simulink model "coaxialQuad_model"  (R2022a)
settings: Solver=VariableStepAuto  StartTime=0.0  StopTime=40  RelTol=1e-3
values from neighbouring files (symbols this model uses):
  Ah = 5,8    [coaxialQuad_init.m]
  Ax = 0    [coaxialQuad_init.m]
  Ay = 0    [coaxialQuad_init.m]
  b = 1.869E-7    (= 1.869e-07)    [coaxialQuad_init.m]
  b_m = 2.415e-6    (= 2.415e-06)    [coaxialQuad_init.m]
  C = 45    [coaxialQuad_init.m]
  d = 1.706E-8    (= 1.706e-08)    [coaxialQuad_init.m]
  Ixx = 0.182    [coaxialQuad_init.m]
  Iyy = 0.188    [coaxialQuad_init.m]
  Izz = 0.335    [coaxialQuad_init.m]
  J = 6.5e-7    (= 6.5e-07)    [coaxialQuad_init.m]
  K_emf = 0.00255    [coaxialQuad_init.m]
  Kt = 0.00255    [coaxialQuad_init.m]
  l = 0.1    [coaxialQuad_init.m]
  L = 1.17e-4    (= 0.000117)    [coaxialQuad_init.m]
  m = 3.1    [coaxialQuad_init.m]
  omega_max = inf    [coaxialQuad_init.m]
  omega_min = 0    [coaxialQuad_init.m]
  phi_D = 0.1    [coaxialQuad_init.m]
  phi_I = 2    [coaxialQuad_init.m]
  phi_P = 2    [coaxialQuad_init.m]
  psi_D = 0    [coaxialQuad_init.m]
  psi_I = 0.1    [coaxialQuad_init.m]
  psi_P = 0.1    [coaxialQuad_init.m]
  R = 0.117    [coaxialQuad_init.m]
  theta_D = 0.1    [coaxialQuad_init.m]
  theta_I = 2    [coaxialQuad_init.m]
  theta_P = 2    [coaxialQuad_init.m]
  V = 16.8    [coaxialQuad_init.m]
  Z_D = 10    [coaxialQuad_init.m]
  Z_I = 5    [coaxialQuad_init.m]
  Z_P = 10    [coaxialQuad_init.m]
undefined symbols (not defined in the file or in its folder): Ion, Lithium
libraries: simulink x17, spsBatteryLib x1, spsControlledCurrentSourceLib x1, spspowerguiLib x1
settings Model: Creator=furkan  LastModifiedBy=Neo
settings DebuggingCC: AlgebraicLoopMsg=none  UnconnectedInputMsg=warning  UnconnectedOutputMsg=warning  UnconnectedLineMsg=warning
settings RTWCC: DLArmComputeVersion=19.05

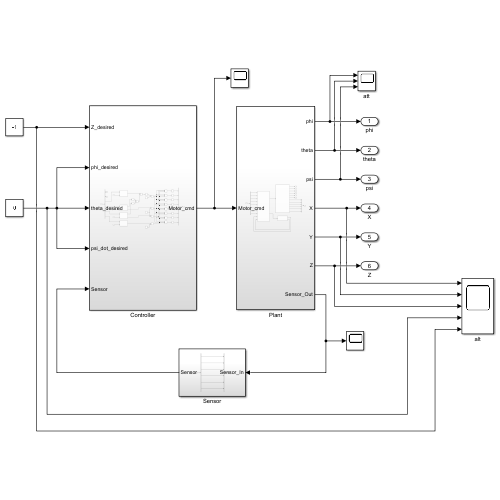
[thumbnail: Simulink's stored preview of the top-level diagram]
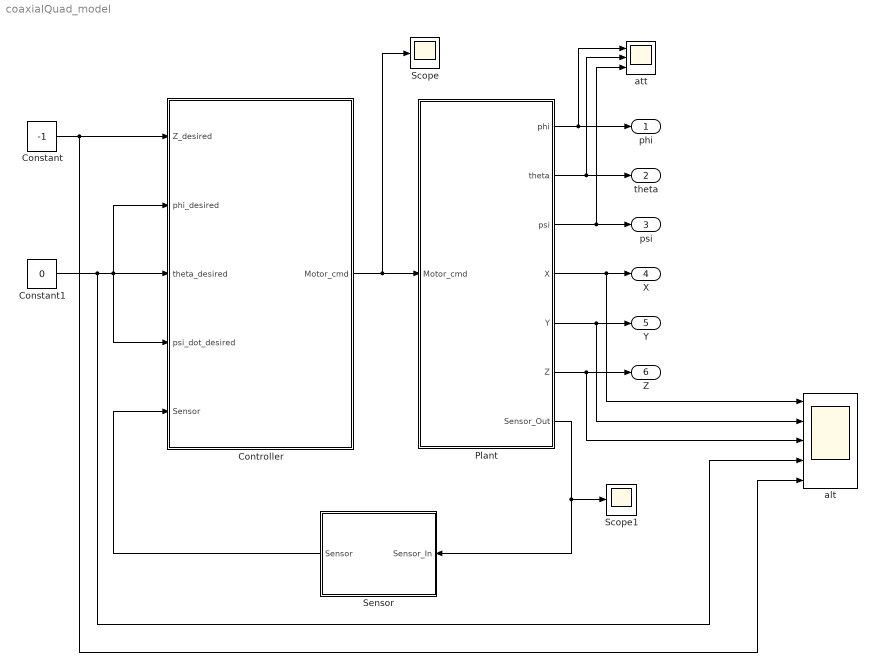
== system coaxialQuad_model ==
  Constant : Constant  Value=-1
  Constant1 : Constant  Value=0
  Controller : Subsystem
  Plant : Subsystem
  Scope : Scope
  Scope1 : Scope
  Sensor : Subsystem
  alt : Scope  NumInputPorts=5
  att : Scope  NumInputPorts=3
  phi : Outport
  theta : Outport  Port=2
  psi : Outport  Port=3
  X : Outport  Port=4
  Y : Outport  Port=5
  Z : Outport  Port=6
  wires:
  Plant/1(phi) -> phi/1, att/1
  Plant/2(theta) -> theta/1, att/2
  Plant/3(psi) -> att/3, psi/1
  Plant/4(X) -> X/1, alt/1
  Plant/5(Y) -> Y/1, alt/2
  Plant/6(Z) -> Z/1, alt/3
  Constant/1 -> Controller/1(Z_desired), alt/5
  Constant1/1 -> Controller/3(theta_desired), Controller/2(phi_desired), Controller/4(psi_dot_desired), alt/4
  Plant/7(Sensor_Out) -> Scope1/1, Sensor/1(Sensor_In)
  Sensor/1(Sensor) -> Controller/5(Sensor)
  Controller/1(Motor_cmd) -> Scope/1, Plant/1(Motor_cmd)

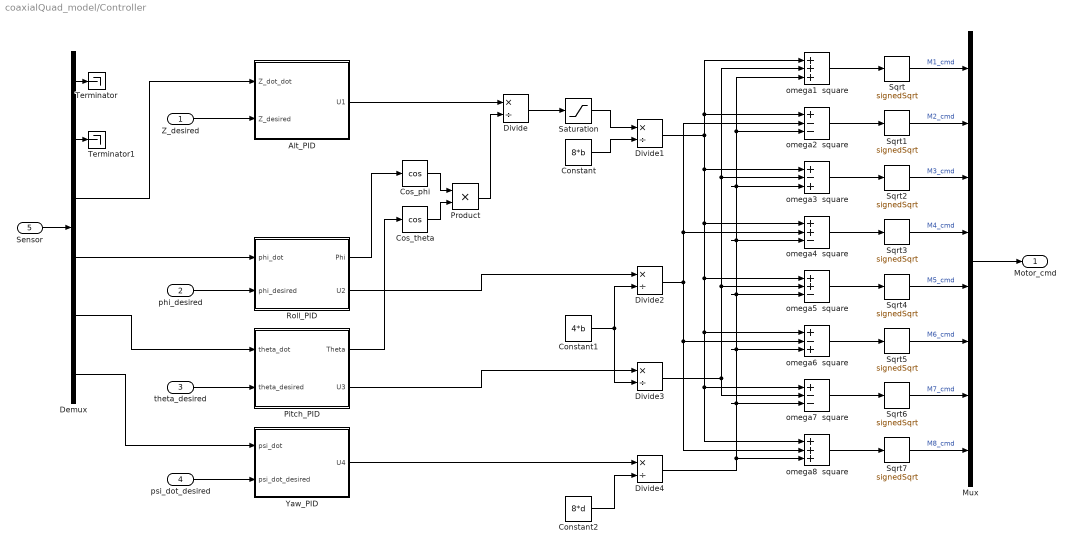
== system coaxialQuad_model/Controller ==
  Z_desired : Inport
  phi_desired : Inport  Port=2
  theta_desired : Inport  Port=3
  psi_dot_desired : Inport  Port=4
  Sensor : Inport  Port=5
  Alt_PID : Subsystem
  Constant : Constant  Value=8*b
  Constant1 : Constant  Value=4*b
  Constant2 : Constant  Value=8*d
  Cos_phi : Trigonometry  Operator=cos
  Cos_theta : Trigonometry  Operator=cos
  Demux : Demux  Outputs=6
  Divide{,1..4} (5 alike) : Product  Inputs=*/  RndMeth=Zero  SaturateOnIntegerOverflow=on
  Mux : Mux  Inputs=8
  Pitch_PID : Subsystem
  Product : Product
  Roll_PID : Subsystem
  Saturation : Saturate  UpperLimit=inf  LowerLimit=0
  Sqrt{,1..7} (8 alike) : Sqrt  Operator=signedSqrt
  Terminator : Terminator
  Terminator1 : Terminator
  Yaw_PID : Subsystem
  omega1  square : Sum  Inputs=+++
  omega2  square : Sum  Inputs=+--
  omega3  square : Sum  Inputs=+-+
  omega4  square : Sum  Inputs=++-
  omega5  square : Sum  Inputs=++-
  omega6  square : Sum  Inputs=+-+
  omega7  square : Sum  Inputs=+--
  omega8  square : Sum  Inputs=+++
  Motor_cmd : Outport
  wires:
  Cos_phi/1 -> Product/1
  Cos_theta/1 -> Product/2
  Product/1 -> Divide/2
  Demux/3 -> Alt_PID/1(Z_dot_dot)
  Z_desired/1 -> Alt_PID/2(Z_desired)
  Alt_PID/1(U1) -> Divide/1
  Divide/1 -> Saturation/1
  Constant/1 -> Divide1/2
  Saturation/1 -> Divide1/1
  Constant1/1 -> Divide3/2, Divide2/2
  Constant2/1 -> Divide4/2
  Demux/4 -> Roll_PID/1(phi_dot)
  phi_desired/1 -> Roll_PID/2(phi_desired)
  Roll_PID/2(U2) -> Divide2/1
  Demux/5 -> Pitch_PID/1(theta_dot)
  theta_desired/1 -> Pitch_PID/2(theta_desired)
  Pitch_PID/2(U3) -> Divide3/1
  Demux/6 -> Yaw_PID/1(psi_dot)
  psi_dot_desired/1 -> Yaw_PID/2(psi_dot_desired)
  Yaw_PID/1(U4) -> Divide4/1
  Divide1/1 -> omega2  square/1, omega1  square/1, omega3  square/1, omega4  square/1, omega5  square/1, omega6  square/1, omega7  square/1, omega8  square/1
  Divide3/1 -> omega7  square/2, omega5  square/2, omega3  square/2, omega1  square/2
  Divide4/1 -> omega8  square/3, omega7  square/3, omega6  square/3, omega5  square/3, omega4  square/3, omega3  square/3, omega1  square/3, omega2  square/3
  omega1  square/1 -> Sqrt/1
  Sqrt/1 -> Mux/1  "M1_cmd"
  Sqrt1/1 -> Mux/2  "M2_cmd"
  omega2  square/1 -> Sqrt1/1
  omega4  square/1 -> Sqrt3/1
  Sqrt3/1 -> Mux/4  "M4_cmd"
  Sqrt2/1 -> Mux/3  "M3_cmd"
  omega3  square/1 -> Sqrt2/1
  omega7  square/1 -> Sqrt6/1
  Sqrt6/1 -> Mux/7  "M7_cmd"
  Sqrt7/1 -> Mux/8  "M8_cmd"
  omega8  square/1 -> Sqrt7/1
  omega6  square/1 -> Sqrt5/1
  Sqrt5/1 -> Mux/6  "M6_cmd"
  Sqrt4/1 -> Mux/5  "M5_cmd"
  omega5  square/1 -> Sqrt4/1
  Divide2/1 -> omega8  square/2, omega6  square/2, omega2  square/2, omega4  square/2
  Demux/1 -> Terminator/1
  Demux/2 -> Terminator1/1
  Sensor/1 -> Demux/1
  Roll_PID/1(Phi) -> Cos_phi/1
  Pitch_PID/1(Theta) -> Cos_theta/1
  Mux/1 -> Motor_cmd/1

== system coaxialQuad_model/Plant ==
  Motor_cmd : Inport
  Battery Plant : Subsystem
  Body Plant : Subsystem
  Demux : Demux  Outputs=8
  Motor Plant : Subsystem
  Mux : Mux  Inputs=6
  phi : Outport
  theta : Outport  Port=2
  psi : Outport  Port=3
  X : Outport  Port=4
  Y : Outport  Port=5
  Z : Outport  Port=6
  Sensor_Out : Outport  Port=7
  wires:
  Body Plant/2(theta) -> theta/1
  Demux/7 -> Motor Plant/7(M7_cmd)  "M7_cmd"
  Demux/1 -> Motor Plant/1(M1_cmd)  "M1_cmd"
  Body Plant/3(psi) -> psi/1
  Body Plant/1(phi) -> phi/1
  Demux/5 -> Motor Plant/5(M5_cmd)  "M5_cmd"
  Demux/2 -> Motor Plant/2(M2_cmd)  "M2_cmd"
  Body Plant/4(X) -> X/1
  Demux/8 -> Motor Plant/8(M8_cmd)  "M8_cmd"
  Body Plant/5(Y) -> Y/1
  Demux/4 -> Motor Plant/4(M4_cmd)  "M4_cmd"
  Body Plant/6(Z) -> Z/1
  Battery Plant/1(Aval_Current) -> Motor Plant/9(Aval_Current)
  Battery Plant/2(Voltage) -> Motor Plant/10(Voltage)
  Demux/6 -> Motor Plant/6(M6_cmd)  "M6_cmd"
  Motor Plant/2(Current) -> Battery Plant/1(Current_draw)
  Demux/3 -> Motor Plant/3(M3_cmd)  "M3_cmd"
  Body Plant/7(X_dot_dot) -> Mux/1  "X_dot_dot"
  Body Plant/8(Y_dot_dot) -> Mux/2  "Y_dot_dot"
  Body Plant/9(Z_dot_dot) -> Mux/3  "Z_dot_dot"
  Body Plant/11(theta_dot) -> Mux/5  "theta_dot"
  Body Plant/12(psi_dot) -> Mux/6  "psi_dot"
  Body Plant/10(phi_dot) -> Mux/4  "phi_dot"
  Mux/1 -> Sensor_Out/1
  Motor_cmd/1 -> Demux/1
  Motor Plant/1(Omegas) -> Body Plant/1(omegas)

== system coaxialQuad_model/Sensor ==
  Sensor_In : Inport
  Demux : Demux  Outputs=6
  Mux : Mux  Inputs=6
  Sensor : Outport
  wires:
  Demux/2 -> Mux/2  "Y_dot_dot"
  Demux/3 -> Mux/3  "Z_dot_dot"
  Demux/6 -> Mux/6  "psi_dot"
  Demux/5 -> Mux/5  "theta_dot"
  Demux/4 -> Mux/4  "phi_dot"
  Demux/1 -> Mux/1  "X_dot_dot"
  Sensor_In/1 -> Demux/1
  Mux/1 -> Sensor/1

== system coaxialQuad_model/Controller/Alt_PID ==
  Z_dot_dot : Inport
  Z_desired : Inport  Port=2
  Add : Sum  Inputs=+-
  Add1 : Sum  Inputs=++-
  Integrator : Integrator
  Integrator1 : Integrator  LimitOutput=on  UpperSaturationLimit=0
  Integrator2 : Integrator
  Z_D : Gain  Gain=Z_D
  Z_I : Gain  Gain=Z_I
  Z_P : Gain  Gain=Z_P
  U1 : Outport
  wires:
  Integrator1/1 -> Add/2
  Z_dot_dot/1 -> Integrator/1
  Z_desired/1 -> Add/1
  Integrator/1 -> Z_D/1, Integrator1/1
  Add/1 -> Z_P/1, Integrator2/1
  Z_I/1 -> Add1/2
  Integrator2/1 -> Z_I/1
  Z_D/1 -> Add1/3
  Z_P/1 -> Add1/1
  Add1/1 -> U1/1

== system coaxialQuad_model/Controller/Pitch_PID ==
  theta_dot : Inport
  theta_desired : Inport  Port=2
  Add4 : Sum  Inputs=+-
  Add5 : Sum  Inputs=++-
  Integrator5 : Integrator  WrapState=on
  Integrator6 : Integrator
  Theta_D : Gain  Gain=theta_D
  Theta_I : Gain  Gain=theta_I
  Theta_P : Gain  Gain=theta_P
  Theta : Outport
  U3 : Outport  Port=2
  wires:
  Theta_D/1 -> Add5/3
  Theta_I/1 -> Add5/2
  theta_dot/1 -> Theta_D/1, Integrator5/1
  Integrator5/1 -> Theta/1, Add4/2
  Add4/1 -> Integrator6/1, Theta_P/1
  Theta_P/1 -> Add5/1
  theta_desired/1 -> Add4/1
  Integrator6/1 -> Theta_I/1
  Add5/1 -> U3/1

== system coaxialQuad_model/Controller/Roll_PID ==
  phi_dot : Inport
  phi_desired : Inport  Port=2
  Add2 : Sum  Inputs=+-
  Add3 : Sum  Inputs=++-
  Integrator3 : Integrator  WrapState=on
  Integrator4 : Integrator
  Phi_D : Gain  Gain=phi_D
  Phi_I : Gain  Gain=phi_I
  Phi_P : Gain  Gain=phi_P
  Phi : Outport
  U2 : Outport  Port=2
  wires:
  phi_desired/1 -> Add2/1
  Integrator3/1 -> Phi/1, Add2/2
  phi_dot/1 -> Phi_D/1, Integrator3/1
  Integrator4/1 -> Phi_I/1
  Add2/1 -> Phi_P/1, Integrator4/1
  Phi_P/1 -> Add3/1
  Phi_I/1 -> Add3/2
  Add3/1 -> U2/1
  Phi_D/1 -> Add3/3

== system coaxialQuad_model/Controller/Yaw_PID ==
  psi_dot : Inport
  psi_dot_desired : Inport  Port=2
  Add6 : Sum  Inputs=-+
  Add7 : Sum  Inputs=+++
  Derivative : Derivative
  Integrator7 : Integrator
  Psi_D : Gain  Gain=psi_D
  Psi_I : Gain  Gain=psi_I
  Psi_P : Gain  Gain=psi_P
  U4 : Outport
  wires:
  Psi_D/1 -> Add7/3
  Psi_I/1 -> Add7/2
  Integrator7/1 -> Psi_I/1
  psi_dot_desired/1 -> Add6/2
  Psi_P/1 -> Add7/1
  Add6/1 -> Derivative/1, Psi_P/1, Integrator7/1
  Derivative/1 -> Psi_D/1
  psi_dot/1 -> Add6/1
  Add7/1 -> U4/1

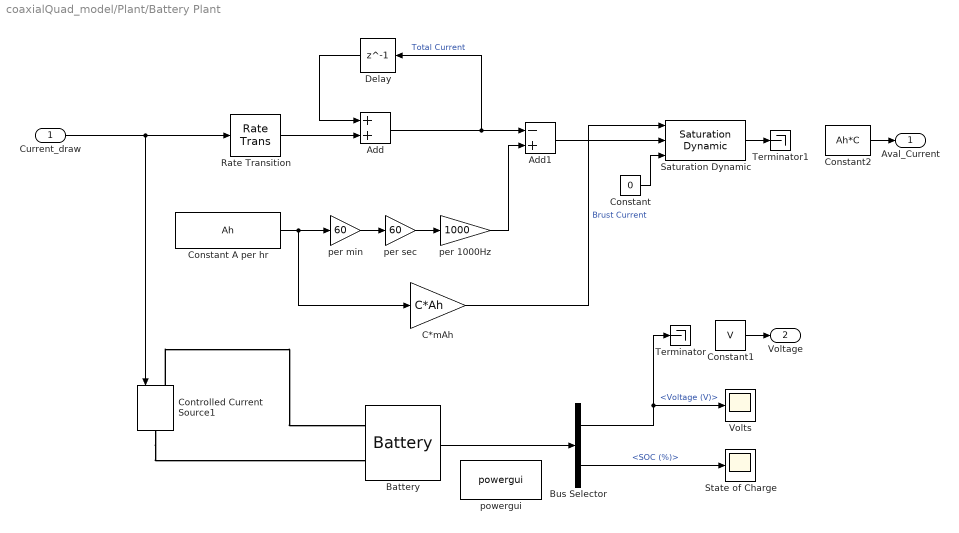
== system coaxialQuad_model/Plant/Battery Plant ==
  Current_draw : Inport
  Add : Sum
  Add1 : Sum  Inputs=-+
  Battery : spsBatteryLib/Battery  BatType=Lithium-Ion  ShowTempParam=off  ThermalPreset=no  ShowAgeParam=off  NomV=V  NomQ=Ah  SOC=100  Batt_Tr=1  PresetModel=on  MaxQ=5  MinV=12.6  FullV=19.555  Dis_rate=2.1739  R=0.0336  Normal_OP=4.5217  expZone="[18.1505     0.245652]"  current=[6.5 13 32.5]  Units=Time  Tci=20  NomT=20  T2=-30  MaxQ2=4.8  FullV2=7.1  Normal_OP2=5.655  expZone2="[6.58           1]"  Rca=0.6  ti=2000  Dp=0  Neq0=0  Tsim=1e6  Ta1=25  Qeol=5.4*0.9  Reol=0.013333*1.2  Char_age=[2.3478, 3]  Dis_age=[2.3478, 10]  N1=1500  N2=10500  N3=1000  N4=1400  Ta2=45  N5=950
  Bus Selector : BusSelector  OutputSignals=Voltage (V),SOC (%)
  C*mAh : Gain  Gain=C*Ah
  Constant : Constant  Value=0
  Constant A per hr : Constant  Value=Ah
  Constant1 : Constant  Value=V
  Constant2 : Constant  Value=Ah*C
  Controlled Current Source1 : spsControlledCurrentSourceLib/Controlled Current Source  Initialize=on  Source_Type=DC  Amplitude=0  Phase=0  Frequency=0  Measurements=None
  Delay : Delay  DelayLength=1
  Rate Transition : RateTransition
  Saturation Dynamic : simulink/Discontinuities/Saturation Dynamic  OutMin=[]  OutMax=[]  OutDataTypeStr=Inherit: Same as second input  OutDataType=fixdt(1, 16)  OutScaling=2^-10  DoSatur=off
  State of Charge : Scope
  Terminator : Terminator
  Terminator1 : Terminator
  Volts : Scope
  per 1000Hz : Gain  Gain=1000
  per min : Gain  Gain=60
  per sec : Gain  Gain=60
  powergui : spspowerguiLib/powergui  Priority=1  SimulationMode=Discrete  SampleTime=0.001  frequency=60  Iterations=50  frequencyindice=0  Pbase=100e6  ErrMax=1e-4  UnitsV=kV  UnitsW=MW  buscounter=0  FunctionMessages=off  echomessages=off  EnableUseOfTLC=off  CurrentSourceSwitches=off  DisableSnubberDevices=off  DisableRonSwitches=off  DisableVfSwitches=off  DisplayEquations=off  AutomaticDiscreteSolvers=off  SolverType=Tustin/Backward Euler (TBE)  Interpol=off  ExternalGateDelay=off  methode=off  Ts=100  x0status=blocks  SPID=on  SwTol=0  HookPort=off  NonlinearTolerance=1e-4  nMaxIteration=100  ContinueOnMaxIteration=off  RestoreLinks=warning  ResistiveCurrentMeasurement=off  Frange=[0:2:500]  Ylog=off  Xlog=on  ShowGrid=off  save=off  variable=ZData  structure=0  ZoomFFT=off  StartTime=0.0  cycles=1  DisplayStyle=1  fundamental=60  FreqAxis=off  MaxFrequency=1000  frequencyindicesteady=1  RmsSteady=1  display=off
  Aval_Current : Outport
  Voltage : Outport  Port=2
  wires:
  Current_draw/1 -> Controlled Current Source1/1, Rate Transition/1
  Rate Transition/1 -> Add/2
  Delay/1 -> Add/1
  Add/1 -> Add1/1, Delay/1  "Total Current"
  Constant A per hr/1 -> C*mAh/1, per min/1
  per min/1 -> per sec/1
  per sec/1 -> per 1000Hz/1
  per 1000Hz/1 -> Add1/2
  Add1/1 -> Saturation Dynamic/2
  C*mAh/1 -> Saturation Dynamic/1  "Brust Current"
  Constant/1 -> Saturation Dynamic/3
  Bus Selector/1 -> Terminator/1, Volts/1  "<Voltage (V)>"
  Bus Selector/2 -> State of Charge/1  "<SOC (%)>"
  Battery/1 -> Bus Selector/1
  Constant2/1 -> Aval_Current/1
  Saturation Dynamic/1 -> Terminator1/1
  Constant1/1 -> Voltage/1
  connections:
  Controlled Current Source1/RConn1 -- Battery/LConn2
  Controlled Current Source1/LConn1 -- Battery/LConn1

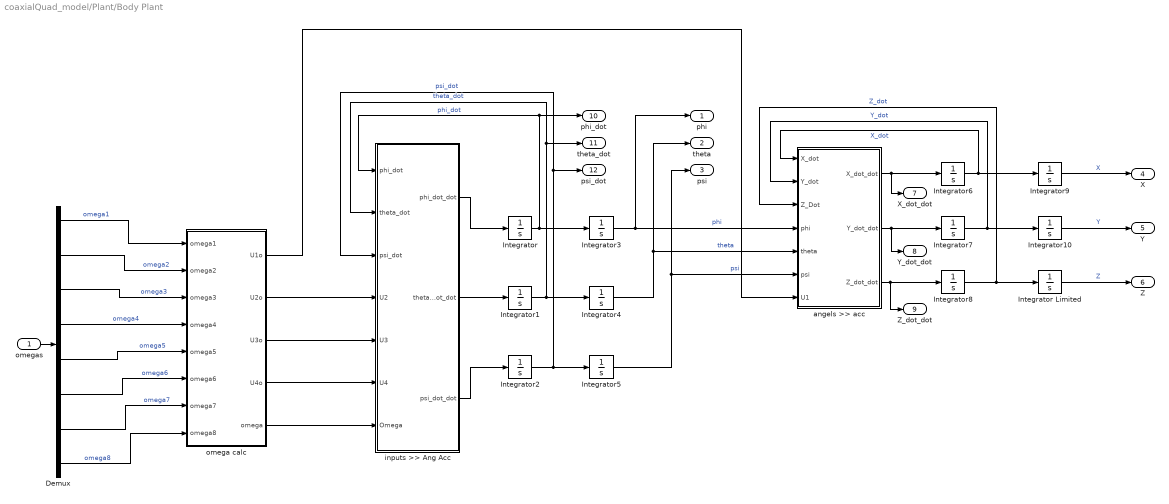
== system coaxialQuad_model/Plant/Body Plant ==
  omegas : Inport
  Demux : Demux  Outputs=8
  Integrator{,1..2,6..10} (8 alike) : Integrator
  Integrator Limited : Integrator  LimitOutput=on  UpperSaturationLimit=0
  Integrator3 : Integrator  WrapState=on
  Integrator4 : Integrator  WrapState=on
  Integrator5 : Integrator  WrapState=on
  angels >> acc : Subsystem
  inputs >> Ang Acc : Subsystem
  omega calc : Subsystem
  phi : Outport
  theta : Outport  Port=2
  psi : Outport  Port=3
  X : Outport  Port=4
  Y : Outport  Port=5
  Z : Outport  Port=6
  X_dot_dot : Outport  Port=7
  Y_dot_dot : Outport  Port=8
  Z_dot_dot : Outport  Port=9
  phi_dot : Outport  Port=10
  theta_dot : Outport  Port=11
  psi_dot : Outport  Port=12
  wires:
  Integrator5/1 -> psi/1, angels >> acc/6(psi)  "psi"
  omega calc/1(U1o) -> angels >> acc/7(U1)
  angels >> acc/1(X_dot_dot) -> X_dot_dot/1, Integrator6/1
  Integrator1/1 -> Integrator4/1, inputs >> Ang Acc/2(theta_dot), theta_dot/1  "theta_dot"
  Integrator2/1 -> Integrator5/1, inputs >> Ang Acc/3(psi_dot), psi_dot/1  "psi_dot"
  Demux/4 -> omega calc/4(omega4)  "omega4"
  Integrator4/1 -> theta/1, angels >> acc/5(theta)  "theta"
  angels >> acc/2(Y_dot_dot) -> Y_dot_dot/1, Integrator7/1
  Demux/6 -> omega calc/6(omega6)  "omega6"
  Integrator10/1 -> Y/1  "Y"
  angels >> acc/3(Z_dot_dot) -> Z_dot_dot/1, Integrator8/1
  Integrator3/1 -> phi/1, angels >> acc/4(phi)  "phi"
  Integrator/1 -> Integrator3/1, inputs >> Ang Acc/1(phi_dot), phi_dot/1  "phi_dot"
  Integrator6/1 -> angels >> acc/1(X_dot), Integrator9/1  "X_dot"
  Demux/2 -> omega calc/2(omega2)  "omega2"
  Integrator Limited/1 -> Z/1  "Z"
  inputs >> Ang Acc/3(psi_dot_dot) -> Integrator2/1
  omega calc/5(omega) -> inputs >> Ang Acc/7(Omega)
  Integrator9/1 -> X/1  "X"
  Integrator8/1 -> Integrator Limited/1, angels >> acc/3(Z_Dot)  "Z_dot"
  Integrator7/1 -> Integrator10/1, angels >> acc/2(Y_dot)  "Y_dot"
  inputs >> Ang Acc/1(phi_dot_dot) -> Integrator/1
  Demux/7 -> omega calc/7(omega7)  "omega7"
  omega calc/4(U4o) -> inputs >> Ang Acc/6(U4)
  omega calc/2(U2o) -> inputs >> Ang Acc/4(U2)
  Demux/8 -> omega calc/8(omega8)  "omega8"
  omega calc/3(U3o) -> inputs >> Ang Acc/5(U3)
  Demux/5 -> omega calc/5(omega5)  "omega5"
  Demux/3 -> omega calc/3(omega3)  "omega3"
  Demux/1 -> omega calc/1(omega1)  "omega1"
  inputs >> Ang Acc/2(theta_dot_dot) -> Integrator1/1
  omegas/1 -> Demux/1

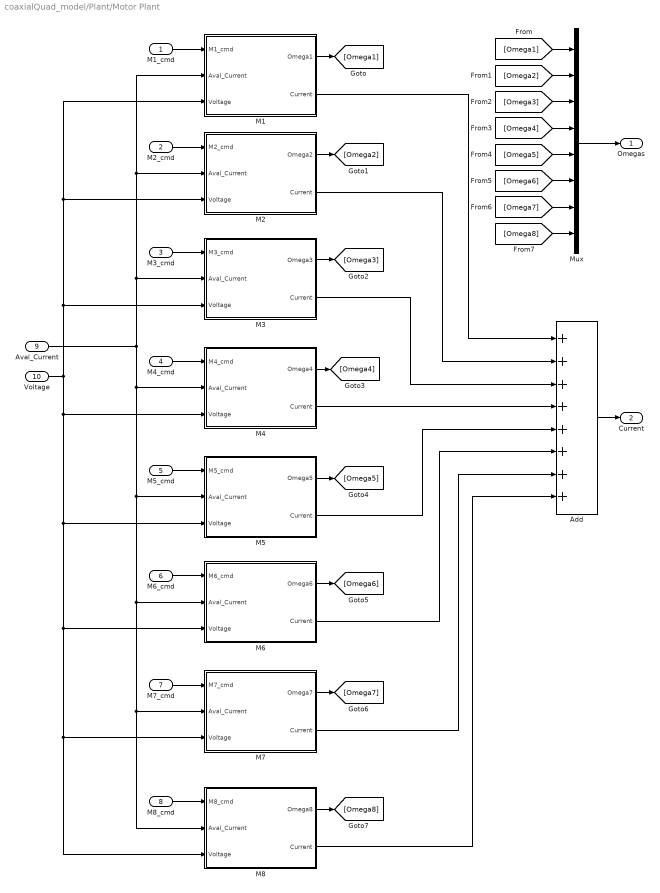
== system coaxialQuad_model/Plant/Motor Plant ==
  M1_cmd : Inport
  M2_cmd : Inport  Port=2
  M3_cmd : Inport  Port=3
  M4_cmd : Inport  Port=4
  M5_cmd : Inport  Port=5
  M6_cmd : Inport  Port=6
  M7_cmd : Inport  Port=7
  M8_cmd : Inport  Port=8
  Aval_Current : Inport  Port=9
  Voltage : Inport  Port=10
  Add : Sum  Inputs=++++++++
  M1 : Subsystem
  M2 : Subsystem
  M3 : Subsystem
  M4 : Subsystem
  M5 : Subsystem
  M6 : Subsystem
  M7 : Subsystem
  M8 : Subsystem
  Mux : Mux  Inputs=8
  Omegas : Outport
  Current : Outport  Port=2
  wires:
  M1_cmd/1 -> M1/1(M1_cmd)
  M2_cmd/1 -> M2/1(M2_cmd)
  M3_cmd/1 -> M3/1(M3_cmd)
  M4_cmd/1 -> M4/1(M4_cmd)
  M6_cmd/1 -> M6/1(M6_cmd)
  Voltage/1 -> M4/3(Voltage), M6/3(Voltage), M7/3(Voltage), M8/3(Voltage), M5/3(Voltage), M1/3(Voltage), M2/3(Voltage), M3/3(Voltage)
  Aval_Current/1 -> M2/2(Aval_Current), M1/2(Aval_Current), M3/2(Aval_Current), M7/2(Aval_Current), M8/2(Aval_Current), M6/2(Aval_Current), M5/2(Aval_Current), M4/2(Aval_Current)
  M8_cmd/1 -> M8/1(M8_cmd)
  M5_cmd/1 -> M5/1(M5_cmd)
  M7_cmd/1 -> M7/1(M7_cmd)
  M1/2(Current) -> Add/1
  M2/2(Current) -> Add/2
  M3/2(Current) -> Add/3
  M4/2(Current) -> Add/4
  M5/2(Current) -> Add/5
  M6/2(Current) -> Add/6
  M7/2(Current) -> Add/7
  M8/2(Current) -> Add/8
  Add/1 -> Current/1
  Mux/1 -> Omegas/1
  M1/1(Omega1) -> [Omega1]
  M2/1(Omega2) -> [Omega2]
  M3/1(Omega3) -> [Omega3]
  M8/1(Omega8) -> [Omega8]
  M7/1(Omega7) -> [Omega7]
  M5/1(Omega5) -> [Omega5]
  M6/1(Omega6) -> [Omega6]
  M4/1(Omega4) -> [Omega4]
  [Omega1] -> Mux/1
  [Omega2] -> Mux/2
  [Omega3] -> Mux/3
  [Omega4] -> Mux/4
  [Omega5] -> Mux/5
  [Omega6] -> Mux/6
  [Omega7] -> Mux/7
  [Omega8] -> Mux/8

== system coaxialQuad_model/Plant/Body Plant/angels >> acc ==
  X_dot : Inport
  Y_dot : Inport  Port=2
  Z_Dot : Inport  Port=3
  phi : Inport  Port=4
  theta : Inport  Port=5
  psi : Inport  Port=6
  U1 : Inport  Port=7
  Divide : Product  Inputs=*/
  Subsystem : Subsystem
  Subsystem1 : Subsystem
  Subsystem2 : Subsystem
  m : Constant  Value=m
  X_dot_dot : Outport
  Y_dot_dot : Outport  Port=2
  Z_dot_dot : Outport  Port=3
  wires:
  U1/1 -> Divide/1
  m/1 -> Divide/2
  X_dot/1 -> Subsystem/1(X_dot)
  phi/1 -> Subsystem2/2(phi), Subsystem1/2(phi), Subsystem/2(phi)
  theta/1 -> Subsystem2/3(theta), Subsystem1/3(theta), Subsystem/3(theta)
  psi/1 -> Subsystem1/4(psi), Subsystem/4(psi)
  Divide/1 -> Subsystem2/4(U1/M), Subsystem1/5(U1/M), Subsystem/5(U1/M)
  Subsystem/1(X_dot_dot) -> X_dot_dot/1
  Y_dot/1 -> Subsystem1/1(Y_dot)
  Z_Dot/1 -> Subsystem2/1(Z_dot)
  Subsystem1/1(Y_dot_dot) -> Y_dot_dot/1
  Subsystem2/1(Z_dot_dot) -> Z_dot_dot/1

== system coaxialQuad_model/Plant/Body Plant/inputs >> Ang Acc ==
  phi_dot : Inport
  theta_dot : Inport  Port=2
  psi_dot : Inport  Port=3
  U2 : Inport  Port=4
  U3 : Inport  Port=5
  U4 : Inport  Port=6
  Omega : Inport  Port=7
  Subsystem : Subsystem
  Subsystem1 : Subsystem
  Subsystem2 : Subsystem
  phi_dot_dot : Outport
  theta_dot_dot : Outport  Port=2
  psi_dot_dot : Outport  Port=3
  wires:
  Subsystem/1(phi_dot_dot) -> phi_dot_dot/1
  Subsystem2/1(psi_dot_dot) -> psi_dot_dot/1
  Subsystem1/1(theta_dot_dot) -> theta_dot_dot/1
  Omega/1 -> Subsystem1/1(Omega), Subsystem/4(Omega)
  psi_dot/1 -> Subsystem/3(psi_dot), Subsystem1/2(psi_dot)
  U3/1 -> Subsystem1/3(U3)
  phi_dot/1 -> Subsystem1/4(phi_dot), Subsystem2/1(phi_dot)
  theta_dot/1 -> Subsystem2/2(Theta_dot), Subsystem/2(theta_dot)
  U2/1 -> Subsystem/1(U2)
  U4/1 -> Subsystem2/3(U4)

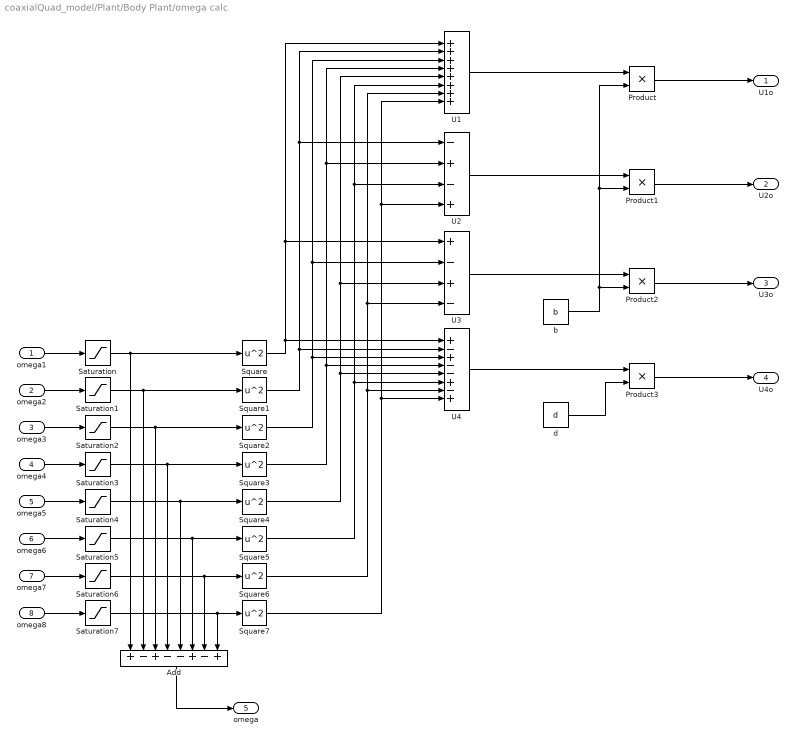
== system coaxialQuad_model/Plant/Body Plant/omega calc ==
  omega1 : Inport
  omega2 : Inport  Port=2
  omega3 : Inport  Port=3
  omega4 : Inport  Port=4
  omega5 : Inport  Port=5
  omega6 : Inport  Port=6
  omega7 : Inport  Port=7
  omega8 : Inport  Port=8
  Add : Sum  Inputs=+-+--+-+
  Product{,1..3} (4 alike) : Product
  Saturation{,1..7} (8 alike) : Saturate  UpperLimit=omega_max  LowerLimit=omega_min
  Square{,1..7} (8 alike) : Math  Operator=square
  U1 : Sum  Inputs=++++++++
  U2 : Sum  Inputs=-+-+
  U3 : Sum  Inputs=+-+-
  U4 : Sum  Inputs=+-+--+-+
  b : Constant  Value=b
  d : Constant  Value=d
  U1o : Outport
  U2o : Outport  Port=2
  U3o : Outport  Port=3
  U4o : Outport  Port=4
  omega : Outport  Port=5
  wires:
  Square6/1 -> U1/7, U3/4, U4/7
  U3/1 -> Product2/1
  omega6/1 -> Saturation5/1
  Square5/1 -> U4/6, U1/6, U2/3
  omega7/1 -> Saturation6/1
  Product2/1 -> U3o/1
  Product1/1 -> U2o/1
  Square4/1 -> U4/5, U1/5, U3/3
  Square3/1 -> U4/4, U1/4, U2/2
  Square/1 -> U4/1, U3/1, U1/1
  b/1 -> Product/2, Product1/2, Product2/2
  omega1/1 -> Saturation/1
  U1/1 -> Product/1
  omega8/1 -> Saturation7/1
  Add/1 -> omega/1
  Square7/1 -> U1/8, U2/4, U4/8
  d/1 -> Product3/2
  omega2/1 -> Saturation1/1
  Square2/1 -> U4/3, U3/2, U1/3
  Product/1 -> U1o/1
  U4/1 -> Product3/1
  Square1/1 -> U4/2, U1/2, U2/1
  omega3/1 -> Saturation2/1
  omega5/1 -> Saturation4/1
  U2/1 -> Product1/1
  omega4/1 -> Saturation3/1
  Product3/1 -> U4o/1
  Saturation/1 -> Square/1, Add/1
  Saturation1/1 -> Add/2, Square1/1
  Saturation2/1 -> Square2/1, Add/3
  Saturation3/1 -> Square3/1, Add/4
  Saturation4/1 -> Add/5, Square4/1
  Saturation5/1 -> Square5/1, Add/6
  Saturation6/1 -> Square6/1, Add/7
  Saturation7/1 -> Add/8, Square7/1

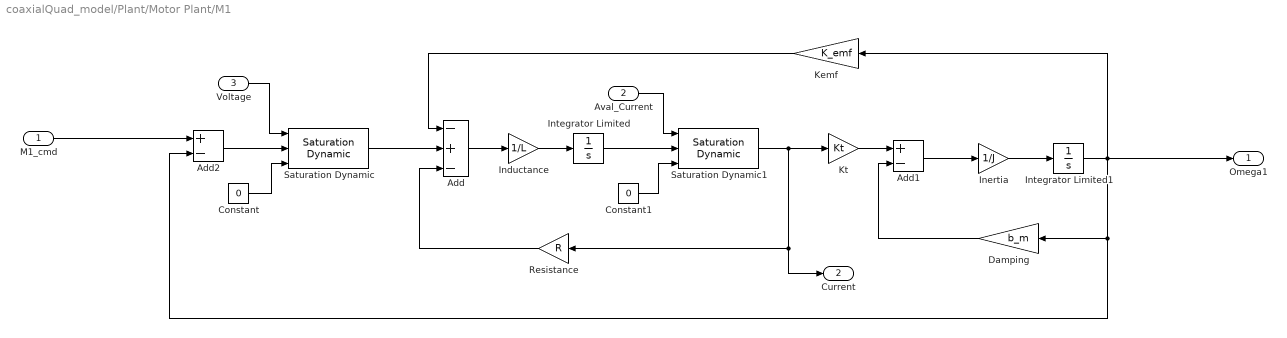
== system coaxialQuad_model/Plant/Motor Plant/M1 ==
  M1_cmd : Inport
  Aval_Current : Inport  Port=2
  Voltage : Inport  Port=3
  Add : Sum  Inputs=-+-
  Add1 : Sum  Inputs=+-
  Add2 : Sum  Inputs=+-
  Constant : Constant  Value=0
  Constant1 : Constant  Value=0
  Damping : Gain  Gain=b_m
  Inductance : Gain  Gain=1/L
  Inertia : Gain  Gain=1/J
  Integrator Limited : Integrator  LimitOutput=on  LowerSaturationLimit=0
  Integrator Limited1 : Integrator  LimitOutput=on  LowerSaturationLimit=0
  Kemf : Gain  Gain=K_emf
  Kt : Gain  Gain=Kt
  Resistance : Gain  Gain=R
  Saturation Dynamic : simulink/Discontinuities/Saturation Dynamic  OutMin=[]  OutMax=[]  OutDataTypeStr=Inherit: Same as second input  OutDataType=fixdt(1, 16)  OutScaling=2^-10  DoSatur=off
  Saturation Dynamic1 : simulink/Discontinuities/Saturation Dynamic  OutMin=[]  OutMax=[]  OutDataTypeStr=Inherit: Same as second input  OutDataType=fixdt(1, 16)  OutScaling=2^-10  DoSatur=off
  Omega1 : Outport
  Current : Outport  Port=2
  wires:
  Add/1 -> Inductance/1
  Saturation Dynamic1/1 -> Current/1, Resistance/1, Kt/1
  Inertia/1 -> Integrator Limited1/1
  M1_cmd/1 -> Add2/1
  Add1/1 -> Inertia/1
  Inductance/1 -> Integrator Limited/1
  Damping/1 -> Add1/2
  Resistance/1 -> Add/3
  Kemf/1 -> Add/1
  Kt/1 -> Add1/1
  Saturation Dynamic/1 -> Add/2
  Add2/1 -> Saturation Dynamic/2
  Integrator Limited/1 -> Saturation Dynamic1/2
  Constant1/1 -> Saturation Dynamic1/3
  Constant/1 -> Saturation Dynamic/3
  Aval_Current/1 -> Saturation Dynamic1/1
  Voltage/1 -> Saturation Dynamic/1
  Integrator Limited1/1 -> Add2/2, Damping/1, Kemf/1, Omega1/1

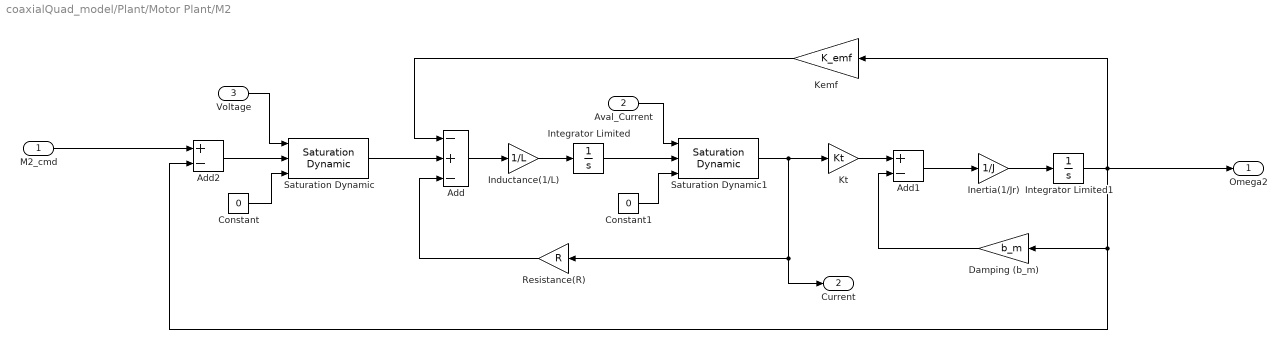
== system coaxialQuad_model/Plant/Motor Plant/M2 ==
  M2_cmd : Inport
  Aval_Current : Inport  Port=2
  Voltage : Inport  Port=3
  Add : Sum  Inputs=-+-
  Add1 : Sum  Inputs=+-
  Add2 : Sum  Inputs=+-
  Constant : Constant  Value=0
  Constant1 : Constant  Value=0
  Damping (b_m) : Gain  Gain=b_m
  Inductance(1/L) : Gain  Gain=1/L
  Inertia(1/Jr) : Gain  Gain=1/J
  Integrator Limited : Integrator  LimitOutput=on  LowerSaturationLimit=0
  Integrator Limited1 : Integrator  LimitOutput=on  LowerSaturationLimit=0
  Kemf : Gain  Gain=K_emf
  Kt : Gain  Gain=Kt
  Resistance(R) : Gain  Gain=R
  Saturation Dynamic : simulink/Discontinuities/Saturation Dynamic  OutMin=[]  OutMax=[]  OutDataTypeStr=Inherit: Same as second input  OutDataType=fixdt(1, 16)  OutScaling=2^-10  DoSatur=off
  Saturation Dynamic1 : simulink/Discontinuities/Saturation Dynamic  OutMin=[]  OutMax=[]  OutDataTypeStr=Inherit: Same as second input  OutDataType=fixdt(1, 16)  OutScaling=2^-10  DoSatur=off
  Omega2 : Outport
  Current : Outport  Port=2
  wires:
  Add/1 -> Inductance(1/L)/1
  Saturation Dynamic1/1 -> Current/1, Resistance(R)/1, Kt/1
  Inertia(1/Jr)/1 -> Integrator Limited1/1
  M2_cmd/1 -> Add2/1
  Integrator Limited1/1 -> Add2/2, Damping (b_m)/1, Kemf/1, Omega2/1
  Add1/1 -> Inertia(1/Jr)/1
  Inductance(1/L)/1 -> Integrator Limited/1
  Damping (b_m)/1 -> Add1/2
  Resistance(R)/1 -> Add/3
  Kemf/1 -> Add/1
  Kt/1 -> Add1/1
  Saturation Dynamic/1 -> Add/2
  Add2/1 -> Saturation Dynamic/2
  Integrator Limited/1 -> Saturation Dynamic1/2
  Constant1/1 -> Saturation Dynamic1/3
  Constant/1 -> Saturation Dynamic/3
  Aval_Current/1 -> Saturation Dynamic1/1
  Voltage/1 -> Saturation Dynamic/1

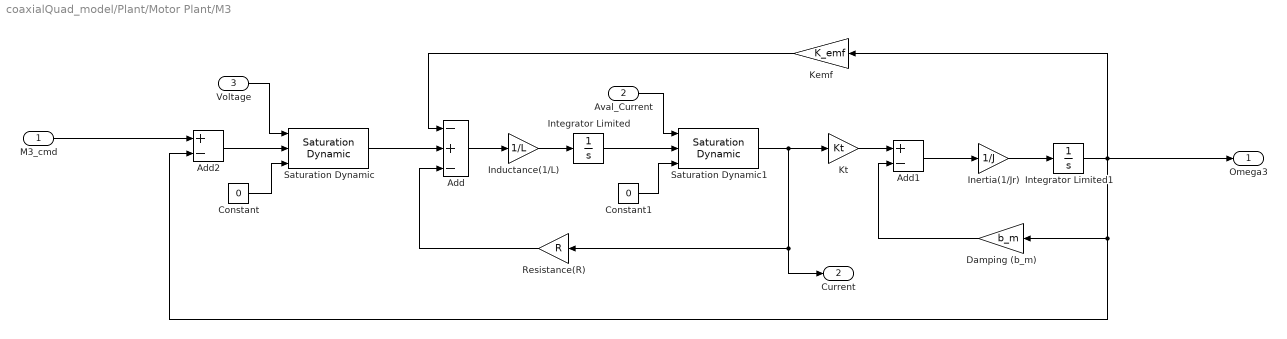
== system coaxialQuad_model/Plant/Motor Plant/M3 ==
  M3_cmd : Inport
  Aval_Current : Inport  Port=2
  Voltage : Inport  Port=3
  Add : Sum  Inputs=-+-
  Add1 : Sum  Inputs=+-
  Add2 : Sum  Inputs=+-
  Constant : Constant  Value=0
  Constant1 : Constant  Value=0
  Damping (b_m) : Gain  Gain=b_m
  Inductance(1/L) : Gain  Gain=1/L
  Inertia(1/Jr) : Gain  Gain=1/J
  Integrator Limited : Integrator  LimitOutput=on  LowerSaturationLimit=0
  Integrator Limited1 : Integrator  LimitOutput=on  LowerSaturationLimit=0
  Kemf : Gain  Gain=K_emf
  Kt : Gain  Gain=Kt
  Resistance(R) : Gain  Gain=R
  Saturation Dynamic : simulink/Discontinuities/Saturation Dynamic  OutMin=[]  OutMax=[]  OutDataTypeStr=Inherit: Same as second input  OutDataType=fixdt(1, 16)  OutScaling=2^-10  DoSatur=off
  Saturation Dynamic1 : simulink/Discontinuities/Saturation Dynamic  OutMin=[]  OutMax=[]  OutDataTypeStr=Inherit: Same as second input  OutDataType=fixdt(1, 16)  OutScaling=2^-10  DoSatur=off
  Omega3 : Outport
  Current : Outport  Port=2
  wires:
  Add/1 -> Inductance(1/L)/1
  Saturation Dynamic1/1 -> Current/1, Resistance(R)/1, Kt/1
  Inertia(1/Jr)/1 -> Integrator Limited1/1
  M3_cmd/1 -> Add2/1
  Integrator Limited1/1 -> Add2/2, Damping (b_m)/1, Kemf/1, Omega3/1
  Add1/1 -> Inertia(1/Jr)/1
  Inductance(1/L)/1 -> Integrator Limited/1
  Damping (b_m)/1 -> Add1/2
  Resistance(R)/1 -> Add/3
  Kemf/1 -> Add/1
  Kt/1 -> Add1/1
  Saturation Dynamic/1 -> Add/2
  Add2/1 -> Saturation Dynamic/2
  Integrator Limited/1 -> Saturation Dynamic1/2
  Constant1/1 -> Saturation Dynamic1/3
  Constant/1 -> Saturation Dynamic/3
  Aval_Current/1 -> Saturation Dynamic1/1
  Voltage/1 -> Saturation Dynamic/1

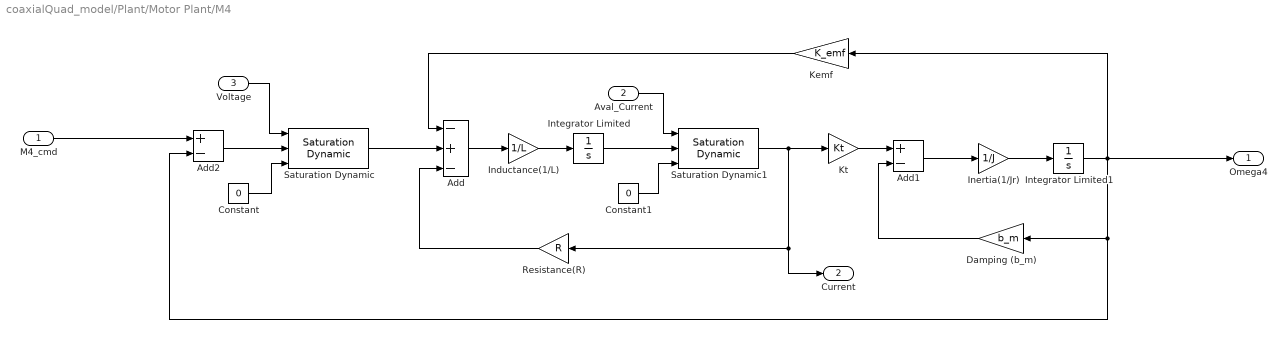
== system coaxialQuad_model/Plant/Motor Plant/M4 ==
  M4_cmd : Inport
  Aval_Current : Inport  Port=2
  Voltage : Inport  Port=3
  Add : Sum  Inputs=-+-
  Add1 : Sum  Inputs=+-
  Add2 : Sum  Inputs=+-
  Constant : Constant  Value=0
  Constant1 : Constant  Value=0
  Damping (b_m) : Gain  Gain=b_m
  Inductance(1/L) : Gain  Gain=1/L
  Inertia(1/Jr) : Gain  Gain=1/J
  Integrator Limited : Integrator  LimitOutput=on  LowerSaturationLimit=0
  Integrator Limited1 : Integrator  LimitOutput=on  LowerSaturationLimit=0
  Kemf : Gain  Gain=K_emf
  Kt : Gain  Gain=Kt
  Resistance(R) : Gain  Gain=R
  Saturation Dynamic : simulink/Discontinuities/Saturation Dynamic  OutMin=[]  OutMax=[]  OutDataTypeStr=Inherit: Same as second input  OutDataType=fixdt(1, 16)  OutScaling=2^-10  DoSatur=off
  Saturation Dynamic1 : simulink/Discontinuities/Saturation Dynamic  OutMin=[]  OutMax=[]  OutDataTypeStr=Inherit: Same as second input  OutDataType=fixdt(1, 16)  OutScaling=2^-10  DoSatur=off
  Omega4 : Outport
  Current : Outport  Port=2
  wires:
  Add/1 -> Inductance(1/L)/1
  Saturation Dynamic1/1 -> Current/1, Resistance(R)/1, Kt/1
  Inertia(1/Jr)/1 -> Integrator Limited1/1
  M4_cmd/1 -> Add2/1
  Integrator Limited1/1 -> Add2/2, Damping (b_m)/1, Kemf/1, Omega4/1
  Add1/1 -> Inertia(1/Jr)/1
  Inductance(1/L)/1 -> Integrator Limited/1
  Damping (b_m)/1 -> Add1/2
  Resistance(R)/1 -> Add/3
  Kemf/1 -> Add/1
  Kt/1 -> Add1/1
  Saturation Dynamic/1 -> Add/2
  Add2/1 -> Saturation Dynamic/2
  Integrator Limited/1 -> Saturation Dynamic1/2
  Constant1/1 -> Saturation Dynamic1/3
  Constant/1 -> Saturation Dynamic/3
  Aval_Current/1 -> Saturation Dynamic1/1
  Voltage/1 -> Saturation Dynamic/1

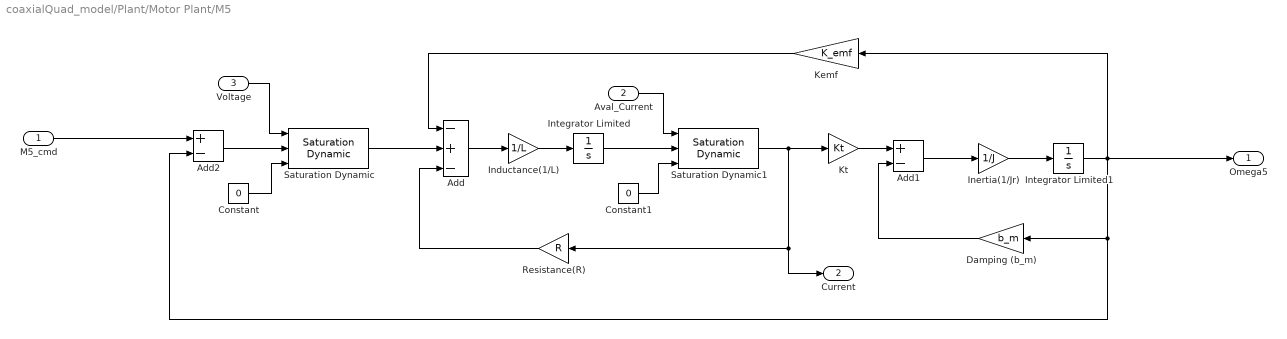
== system coaxialQuad_model/Plant/Motor Plant/M5 ==
  M5_cmd : Inport
  Aval_Current : Inport  Port=2
  Voltage : Inport  Port=3
  Add : Sum  Inputs=-+-
  Add1 : Sum  Inputs=+-
  Add2 : Sum  Inputs=+-
  Constant : Constant  Value=0
  Constant1 : Constant  Value=0
  Damping (b_m) : Gain  Gain=b_m
  Inductance(1/L) : Gain  Gain=1/L
  Inertia(1/Jr) : Gain  Gain=1/J
  Integrator Limited : Integrator  LimitOutput=on  LowerSaturationLimit=0
  Integrator Limited1 : Integrator  LimitOutput=on  LowerSaturationLimit=0
  Kemf : Gain  Gain=K_emf
  Kt : Gain  Gain=Kt
  Resistance(R) : Gain  Gain=R
  Saturation Dynamic : simulink/Discontinuities/Saturation Dynamic  OutMin=[]  OutMax=[]  OutDataTypeStr=Inherit: Same as second input  OutDataType=fixdt(1, 16)  OutScaling=2^-10  DoSatur=off
  Saturation Dynamic1 : simulink/Discontinuities/Saturation Dynamic  OutMin=[]  OutMax=[]  OutDataTypeStr=Inherit: Same as second input  OutDataType=fixdt(1, 16)  OutScaling=2^-10  DoSatur=off
  Omega5 : Outport
  Current : Outport  Port=2
  wires:
  Add/1 -> Inductance(1/L)/1
  Saturation Dynamic1/1 -> Current/1, Resistance(R)/1, Kt/1
  Inertia(1/Jr)/1 -> Integrator Limited1/1
  M5_cmd/1 -> Add2/1
  Integrator Limited1/1 -> Add2/2, Damping (b_m)/1, Kemf/1, Omega5/1
  Add1/1 -> Inertia(1/Jr)/1
  Inductance(1/L)/1 -> Integrator Limited/1
  Damping (b_m)/1 -> Add1/2
  Resistance(R)/1 -> Add/3
  Kemf/1 -> Add/1
  Kt/1 -> Add1/1
  Saturation Dynamic/1 -> Add/2
  Add2/1 -> Saturation Dynamic/2
  Integrator Limited/1 -> Saturation Dynamic1/2
  Constant1/1 -> Saturation Dynamic1/3
  Constant/1 -> Saturation Dynamic/3
  Aval_Current/1 -> Saturation Dynamic1/1
  Voltage/1 -> Saturation Dynamic/1

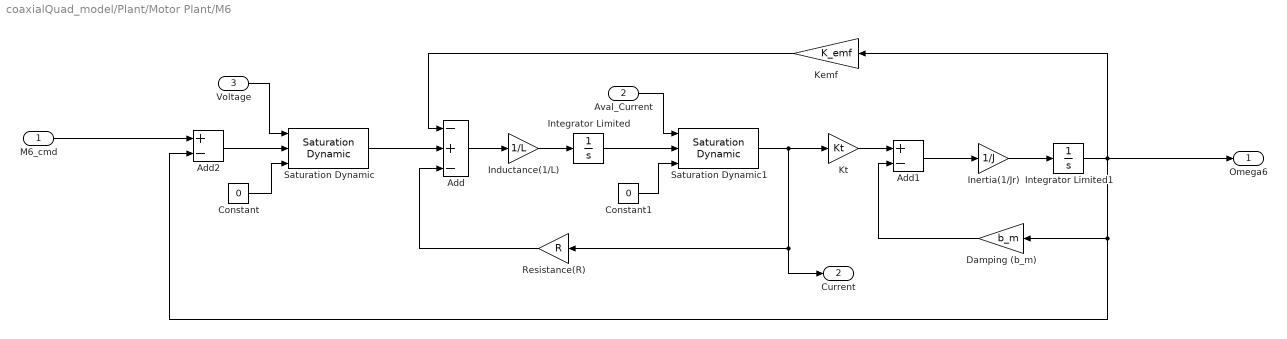
== system coaxialQuad_model/Plant/Motor Plant/M6 ==
  M6_cmd : Inport
  Aval_Current : Inport  Port=2
  Voltage : Inport  Port=3
  Add : Sum  Inputs=-+-
  Add1 : Sum  Inputs=+-
  Add2 : Sum  Inputs=+-
  Constant : Constant  Value=0
  Constant1 : Constant  Value=0
  Damping (b_m) : Gain  Gain=b_m
  Inductance(1/L) : Gain  Gain=1/L
  Inertia(1/Jr) : Gain  Gain=1/J
  Integrator Limited : Integrator  LimitOutput=on  LowerSaturationLimit=0
  Integrator Limited1 : Integrator  LimitOutput=on  LowerSaturationLimit=0
  Kemf : Gain  Gain=K_emf
  Kt : Gain  Gain=Kt
  Resistance(R) : Gain  Gain=R
  Saturation Dynamic : simulink/Discontinuities/Saturation Dynamic  OutMin=[]  OutMax=[]  OutDataTypeStr=Inherit: Same as second input  OutDataType=fixdt(1, 16)  OutScaling=2^-10  DoSatur=off
  Saturation Dynamic1 : simulink/Discontinuities/Saturation Dynamic  OutMin=[]  OutMax=[]  OutDataTypeStr=Inherit: Same as second input  OutDataType=fixdt(1, 16)  OutScaling=2^-10  DoSatur=off
  Omega6 : Outport
  Current : Outport  Port=2
  wires:
  Add/1 -> Inductance(1/L)/1
  Saturation Dynamic1/1 -> Current/1, Resistance(R)/1, Kt/1
  Inertia(1/Jr)/1 -> Integrator Limited1/1
  M6_cmd/1 -> Add2/1
  Integrator Limited1/1 -> Add2/2, Damping (b_m)/1, Kemf/1, Omega6/1
  Add1/1 -> Inertia(1/Jr)/1
  Inductance(1/L)/1 -> Integrator Limited/1
  Damping (b_m)/1 -> Add1/2
  Resistance(R)/1 -> Add/3
  Kemf/1 -> Add/1
  Kt/1 -> Add1/1
  Saturation Dynamic/1 -> Add/2
  Add2/1 -> Saturation Dynamic/2
  Integrator Limited/1 -> Saturation Dynamic1/2
  Constant1/1 -> Saturation Dynamic1/3
  Constant/1 -> Saturation Dynamic/3
  Aval_Current/1 -> Saturation Dynamic1/1
  Voltage/1 -> Saturation Dynamic/1

== system coaxialQuad_model/Plant/Motor Plant/M7 ==
  M7_cmd : Inport
  Aval_Current : Inport  Port=2
  Voltage : Inport  Port=3
  Add : Sum  Inputs=-+-
  Add1 : Sum  Inputs=+-
  Add2 : Sum  Inputs=+-
  Constant : Constant  Value=0
  Constant1 : Constant  Value=0
  Damping (b_m) : Gain  Gain=b_m
  Inductance(1/L) : Gain  Gain=1/L
  Inertia(1/Jr) : Gain  Gain=1/J
  Integrator Limited : Integrator  LimitOutput=on  LowerSaturationLimit=0
  Integrator Limited1 : Integrator  LimitOutput=on  LowerSaturationLimit=0
  Kemf : Gain  Gain=K_emf
  Kt : Gain  Gain=Kt
  Resistance(R) : Gain  Gain=R
  Saturation Dynamic : simulink/Discontinuities/Saturation Dynamic  OutMin=[]  OutMax=[]  OutDataTypeStr=Inherit: Same as second input  OutDataType=fixdt(1, 16)  OutScaling=2^-10  DoSatur=off
  Saturation Dynamic1 : simulink/Discontinuities/Saturation Dynamic  OutMin=[]  OutMax=[]  OutDataTypeStr=Inherit: Same as second input  OutDataType=fixdt(1, 16)  OutScaling=2^-10  DoSatur=off
  Omega7 : Outport
  Current : Outport  Port=2
  wires:
  Add/1 -> Inductance(1/L)/1
  Saturation Dynamic1/1 -> Current/1, Resistance(R)/1, Kt/1
  Inertia(1/Jr)/1 -> Integrator Limited1/1
  M7_cmd/1 -> Add2/1
  Integrator Limited1/1 -> Add2/2, Damping (b_m)/1, Kemf/1, Omega7/1
  Add1/1 -> Inertia(1/Jr)/1
  Inductance(1/L)/1 -> Integrator Limited/1
  Damping (b_m)/1 -> Add1/2
  Resistance(R)/1 -> Add/3
  Kemf/1 -> Add/1
  Kt/1 -> Add1/1
  Saturation Dynamic/1 -> Add/2
  Add2/1 -> Saturation Dynamic/2
  Integrator Limited/1 -> Saturation Dynamic1/2
  Constant1/1 -> Saturation Dynamic1/3
  Constant/1 -> Saturation Dynamic/3
  Aval_Current/1 -> Saturation Dynamic1/1
  Voltage/1 -> Saturation Dynamic/1

== system coaxialQuad_model/Plant/Motor Plant/M8 ==
  M8_cmd : Inport
  Aval_Current : Inport  Port=2
  Voltage : Inport  Port=3
  Add : Sum  Inputs=-+-
  Add1 : Sum  Inputs=+-
  Add2 : Sum  Inputs=+-
  Constant : Constant  Value=0
  Constant1 : Constant  Value=0
  Damping (b_m) : Gain  Gain=b_m
  Inductance(1/L) : Gain  Gain=1/L
  Inertia(1/Jr) : Gain  Gain=1/J
  Integrator Limited : Integrator  LimitOutput=on  LowerSaturationLimit=0
  Integrator Limited1 : Integrator  LimitOutput=on  LowerSaturationLimit=0
  Kemf : Gain  Gain=K_emf
  Kt : Gain  Gain=Kt
  Resistance(R) : Gain  Gain=R
  Saturation Dynamic : simulink/Discontinuities/Saturation Dynamic  OutMin=[]  OutMax=[]  OutDataTypeStr=Inherit: Same as second input  OutDataType=fixdt(1, 16)  OutScaling=2^-10  DoSatur=off
  Saturation Dynamic1 : simulink/Discontinuities/Saturation Dynamic  OutMin=[]  OutMax=[]  OutDataTypeStr=Inherit: Same as second input  OutDataType=fixdt(1, 16)  OutScaling=2^-10  DoSatur=off
  Omega8 : Outport
  Current : Outport  Port=2
  wires:
  Add/1 -> Inductance(1/L)/1
  Saturation Dynamic1/1 -> Current/1, Resistance(R)/1, Kt/1
  Inertia(1/Jr)/1 -> Integrator Limited1/1
  M8_cmd/1 -> Add2/1
  Integrator Limited1/1 -> Add2/2, Damping (b_m)/1, Kemf/1, Omega8/1
  Add1/1 -> Inertia(1/Jr)/1
  Inductance(1/L)/1 -> Integrator Limited/1
  Damping (b_m)/1 -> Add1/2
  Resistance(R)/1 -> Add/3
  Kemf/1 -> Add/1
  Kt/1 -> Add1/1
  Saturation Dynamic/1 -> Add/2
  Add2/1 -> Saturation Dynamic/2
  Integrator Limited/1 -> Saturation Dynamic1/2
  Constant1/1 -> Saturation Dynamic1/3
  Constant/1 -> Saturation Dynamic/3
  Aval_Current/1 -> Saturation Dynamic1/1
  Voltage/1 -> Saturation Dynamic/1

== system coaxialQuad_model/Plant/Body Plant/angels >> acc/Subsystem ==
  X_dot : Inport
  phi : Inport  Port=2
  theta : Inport  Port=3
  psi : Inport  Port=4
  U1/M : Inport  Port=5
  Add : Sum
  Add1 : Sum  Inputs=+-
  Ax/m : Constant  Value=Ax/m
  Cos : Trigonometry  Operator=cos
  Cos1 : Trigonometry  Operator=cos
  Product : Product
  Product1 : Product
  Product2 : Product  Inputs=3
  Product3 : Product
  Sin : Trigonometry
  Sin1 : Trigonometry
  Sin2 : Trigonometry
  X_dot_dot : Outport
  wires:
  U1/M/1 -> Product/1
  phi/1 -> Cos/1, Sin/1
  psi/1 -> Sin1/1, Cos1/1
  theta/1 -> Sin2/1
  Sin/1 -> Product1/1
  Sin1/1 -> Product1/2
  Cos/1 -> Product2/1
  Cos1/1 -> Product2/2
  Sin2/1 -> Product2/3
  Product1/1 -> Add/1
  Product2/1 -> Add/2
  Add/1 -> Product/2
  X_dot/1 -> Product3/1
  Ax/m/1 -> Product3/2
  Product/1 -> Add1/1
  Product3/1 -> Add1/2
  Add1/1 -> X_dot_dot/1

== system coaxialQuad_model/Plant/Body Plant/angels >> acc/Subsystem1 ==
  Y_dot : Inport
  phi : Inport  Port=2
  theta : Inport  Port=3
  psi : Inport  Port=4
  U1/M : Inport  Port=5
  Add : Sum  Inputs=-+
  Add1 : Sum  Inputs=+-
  Ay/m : Constant  Value=Ay/m
  Cos : Trigonometry  Operator=cos
  Cos1 : Trigonometry  Operator=cos
  Product : Product
  Product1 : Product
  Product2 : Product  Inputs=3
  Product3 : Product
  Sin : Trigonometry
  Sin1 : Trigonometry
  Sin2 : Trigonometry
  Y_dot_dot : Outport
  wires:
  U1/M/1 -> Product/1
  phi/1 -> Cos/1, Sin/1
  psi/1 -> Sin1/1, Cos1/1
  theta/1 -> Sin2/1
  Sin/1 -> Product1/1
  Cos/1 -> Product2/1
  Sin2/1 -> Product2/3
  Product1/1 -> Add/1
  Product2/1 -> Add/2
  Add/1 -> Product/2
  Y_dot/1 -> Product3/1
  Ay/m/1 -> Product3/2
  Product/1 -> Add1/1
  Product3/1 -> Add1/2
  Add1/1 -> Y_dot_dot/1
  Cos1/1 -> Product1/2
  Sin1/1 -> Product2/2

== system coaxialQuad_model/Plant/Body Plant/angels >> acc/Subsystem2 ==
  Z_dot : Inport
  phi : Inport  Port=2
  theta : Inport  Port=3
  U1/M : Inport  Port=4
  Add : Sum  Inputs=-+
  Add1 : Sum  Inputs=+-
  Ay/m : Constant  Value=Ay/m
  Cos : Trigonometry  Operator=cos
  Product2 : Product  Inputs=3
  Product3 : Product
  Sin2 : Trigonometry  Operator=cos
  g : Constant  Value=9.81
  Z_dot_dot : Outport
  wires:
  phi/1 -> Cos/1
  theta/1 -> Sin2/1
  Sin2/1 -> Product2/3
  g/1 -> Add/1
  Product2/1 -> Add/2
  Z_dot/1 -> Product3/1
  Ay/m/1 -> Product3/2
  Add/1 -> Add1/1
  Product3/1 -> Add1/2
  Add1/1 -> Z_dot_dot/1
  Cos/1 -> Product2/2
  U1/M/1 -> Product2/1

== system coaxialQuad_model/Plant/Body Plant/inputs >> Ang Acc/Subsystem ==
  U2 : Inport
  theta_dot : Inport  Port=2
  psi_dot : Inport  Port=3
  Omega : Inport  Port=4
  Add : Sum  Inputs=+++
  Divide : Product  Inputs=*/
  I : Constant  Value=l
  Ixx : Constant  Value=Ixx
  Iyy-Izz : Constant  Value=Iyy-Izz
  Jr : Constant  Value=J
  Product : Product
  Product1 : Product  Inputs=3
  Product2 : Product  Inputs=3
  phi_dot_dot : Outport
  wires:
  Iyy-Izz/1 -> Product2/3
  Add/1 -> Divide/1
  I/1 -> Product/1
  theta_dot/1 -> Product1/3, Product2/1
  Product2/1 -> Add/3
  Product1/1 -> Add/2
  Ixx/1 -> Divide/2
  U2/1 -> Product/2
  Jr/1 -> Product1/1
  Product/1 -> Add/1
  Divide/1 -> phi_dot_dot/1
  Omega/1 -> Product1/2
  psi_dot/1 -> Product2/2

== system coaxialQuad_model/Plant/Body Plant/inputs >> Ang Acc/Subsystem1 ==
  Omega : Inport
  psi_dot : Inport  Port=2
  U3 : Inport  Port=3
  phi_dot : Inport  Port=4
  Add : Sum  Inputs=+-+
  Divide : Product  Inputs=*/
  I : Constant  Value=l
  Iyy : Constant  Value=Iyy
  Izz-Ixx : Constant  Value=Izz-Ixx
  Jr : Constant  Value=J
  Product : Product
  Product1 : Product  Inputs=3
  Product2 : Product  Inputs=3
  theta_dot_dot : Outport
  wires:
  Izz-Ixx/1 -> Product2/3
  Add/1 -> Divide/1
  I/1 -> Product/1
  phi_dot/1 -> Product1/3, Product2/1
  Product2/1 -> Add/3
  Product1/1 -> Add/2
  Iyy/1 -> Divide/2
  U3/1 -> Product/2
  Jr/1 -> Product1/1
  Product/1 -> Add/1
  Divide/1 -> theta_dot_dot/1
  Omega/1 -> Product1/2
  psi_dot/1 -> Product2/2

== system coaxialQuad_model/Plant/Body Plant/inputs >> Ang Acc/Subsystem2 ==
  phi_dot : Inport
  Theta_dot : Inport  Port=2
  U4 : Inport  Port=3
  Add : Sum
  Divide : Product  Inputs=*/
  Ixx-Iyy : Constant  Value=Ixx-Iyy
  Izz : Constant  Value=Izz
  Product : Product  Inputs=3
  psi_dot_dot : Outport
  wires:
  Product/1 -> Add/2
  Divide/1 -> psi_dot_dot/1
  Add/1 -> Divide/1
  Izz/1 -> Divide/2
  U4/1 -> Add/1
  Ixx-Iyy/1 -> Product/3
  phi_dot/1 -> Product/2
  Theta_dot/1 -> Product/1
